simulink model "SimulationBlock"  (R2019b)
settings: Solver=ode23tb  StartTime=0.0  StopTime=100  RelTol=1e-3
values from neighbouring files (symbols this model uses):
  Sys = SymbolicSolver(Sys)    [TestBuild_v1.m]
settings Model: Creator=aksland2  LastModifiedBy=aksland2

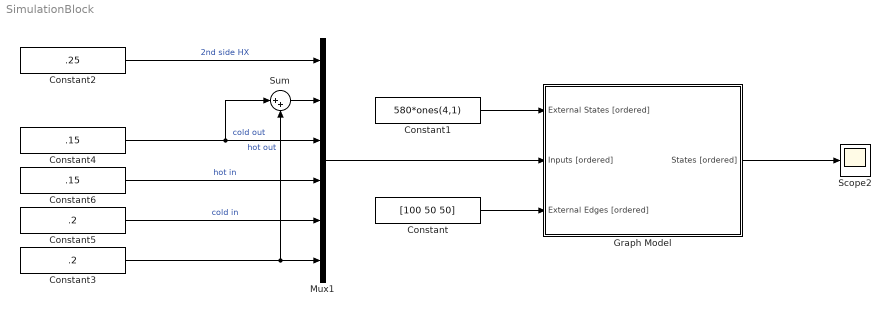
== system SimulationBlock ==
  Constant : Constant  Value=[100 50 50]
  Constant1 : Constant  Value=580*ones(4,1)
  Constant2 : Constant  Value=.25
  Constant3 : Constant  Value=.2
  Constant4 : Constant  Value=.15
  Constant5 : Constant  Value=.2
  Constant6 : Constant  Value=.15
  Graph Model : Subsystem  mask{Sys=Sys}
      mask prompts: Sys "Graph Model"
  Mux1 : Mux  Inputs=6
  Scope2 : Scope
  Sum : Sum  Inputs=|++
  wires:
  Constant2/1 -> Mux1/1  "2nd side HX"
  Constant3/1 -> Sum/2, Mux1/6  "hot out"
  Constant4/1 -> Sum/1, Mux1/3  "cold out"
  Constant5/1 -> Mux1/5  "cold in"
  Constant6/1 -> Mux1/4  "hot in"
  Sum/1 -> Mux1/2
  Constant1/1 -> Graph Model/1(External States [ordered])
  Mux1/1 -> Graph Model/2(Inputs [ordered])
  Constant/1 -> Graph Model/3(External Edges [ordered])
  Graph Model/1(States [ordered]) -> Scope2/1

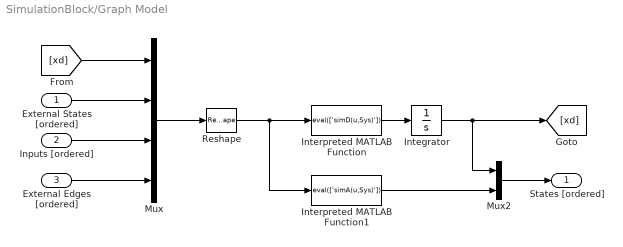
== system SimulationBlock/Graph Model ==
  External States [ordered] : Inport
  Inputs [ordered] : Inport  Port=2
  External Edges [ordered] : Inport  Port=3
  Integrator : Integrator  InitialCondition=Sys.x_init(1:4)
  Interpreted MATLAB Function : MATLABFcn  MATLABFcn=eval(['simD(u,Sys)'])  OutputDimensions=4
  Interpreted MATLAB Function1 : MATLABFcn  MATLABFcn=eval(['simA(u,Sys)'])  OutputDimensions=5
  Mux : Mux
  Mux2 : Mux  Inputs=2
  Reshape : Reshape
  States [ordered] : Outport
  wires:
  Inputs [ordered]/1 -> Mux/3
  External Edges [ordered]/1 -> Mux/4
  Interpreted MATLAB Function1/1 -> Mux2/2
  Integrator/1 -> [xd], Mux2/1
  Interpreted MATLAB Function/1 -> Integrator/1
  Mux/1 -> Reshape/1
  External States [ordered]/1 -> Mux/2
  Reshape/1 -> Interpreted MATLAB Function/1, Interpreted MATLAB Function1/1
  [xd] -> Mux/1
  Mux2/1 -> States [ordered]/1
